simulink model "SimplePendulumWithFeedback"  (Simulink 7.7)
settings: Solver=ode45  StartTime=0.0  StopTime=T  RelTol=1e-3
values from neighbouring files (symbols this model uses):
  b = 1    [pendulum.m]    (also in pendulum1.m = 0.5; pendulum2.m = 0; pendulum3.m = 0; pendulum4.m = 0)
  den = ctr.den{1}    [car1.m]    (also in car2.m; car3.m; car4.m; pendulum.m)
  g = 9.8    [pendulum.m]    (also in pendulum1.m; pendulum2.m; pendulum3.m; pendulum4.m)
  J = mp*l^2/12    (= 0.00375)    [pendulum.m]    (also in pendulum1.m; pendulum2.m; pendulum3.m; pendulum4.m)
  l = 0.3    [pendulum.m]    (also in pendulum1.m; pendulum2.m; pendulum3.m; pendulum4.m)
  mp = 0.5    [pendulum.m]    (also in pendulum1.m; pendulum2.m; pendulum3.m; pendulum4.m)
  num = ctr.num{1}    [car1.m]    (also in car2.m; car3.m; car4.m; pendulum.m = K * ctr.num{1})
  r = l/2    (= 0.15)    [pendulum1.m]    (also in pendulum2.m; pendulum3.m; pendulum4.m; pendulum5.m)
  theta0 = pi - pi/8    (= 2.74889357189)    [pendulum.m]    (also in pendulum1.m = 3.09159265359; pendulum2.m = 1.57079632679; pendulum3.m = 1.57079632679; pendulum4.m = 1.57079632679)
  thetaBar = pi    (= 3.14159265359)    [pendulum.m]    (also in pendulum2.m; pendulum3.m; pendulum4.m = 2.35619449019; pendulum5.m = 2.35619449019)
settings Model: Creator=mauricio  LastModifiedBy=mauricio
settings DebuggingCC: SolverPrmCheckMsg=none

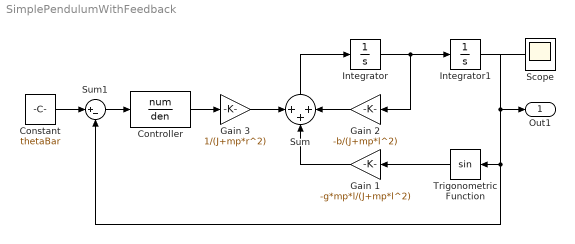
== system SimplePendulumWithFeedback ==
  Constant : Constant  Value=thetaBar
  Controller : TransferFcn  Numerator=num  Denominator=den
  Gain 1 : Gain  Gain=-g*mp*l/(J+mp*l^2)
  Gain 2 : Gain  Gain=-b/(J+mp*l^2)
  Gain 3 : Gain  Gain=1/(J+mp*r^2)
  Integrator : Integrator
  Integrator1 : Integrator  InitialCondition=theta0
  Scope : Scope
      settings: YMin=-3.141592653589793  YMax=3.141592653589793
  Sum : Sum  Inputs=+++
  Sum1 : Sum  Inputs=|+-
  Trigonometric Function : Trigonometry
  Out1 : Outport
  wires:
  Integrator/1 -> Integrator1/1, Gain 2/1
  Integrator1/1 -> Scope/1, Trigonometric Function/1, Sum1/2, Out1/1
  Trigonometric Function/1 -> Gain 1/1
  Sum/1 -> Integrator/1
  Gain 2/1 -> Sum/3
  Gain 1/1 -> Sum/2
  Sum1/1 -> Controller/1
  Controller/1 -> Gain 3/1
  Constant/1 -> Sum1/1
  Gain 3/1 -> Sum/1
